simulink model "gm_uz_endat_interface_2025b"  (R2025b)
settings: Solver=FixedStepDiscrete  StartTime=0.0  StopTime=1.3e-3  RelTol=1e-3
undefined symbols (not defined in the file or in its folder): binary_or_gray, bit_sum, delay_first_clk_on_off, endat_clk_divider, endat_encoder_bit_width_multi_turn, endat_encoder_bit_width_single_turn, endat_encoder_number_of_CRC_bits, f_ADC, f_clock, PLL, t_ADC, t_clock, XData
libraries: hdlmdlgenlib x123, simulink x35, hdlsllib x29, simulink_extras x13
(part 3 of 4)

== system gm_uz_endat_interface_2025b/uz_endat_interface/position_to_speed_pll/Sine HDL Optimized1 ==
  u : Inport  OutDataTypeStr=fixdt(1, 27, 20)  SampleTime=1e-08
  sincos hdl : Subsystem  mask{NumDataPoints=256, TableDataTypeStr=fixdt(0,26,20), SimulateLUTROMDelay='Off'}
      mask prompts: NumDataPoints "HDLShared:hdlshared:CosineHDL_Npts"; TableDataTypeStr "Simulink:blkprm_prompts:TABLE_UNIFIEDDATATYPE"; SimulateLUTROMDelay "HDLShared:hdlshared:CosineHDL_SimulateLUTDelay"
      mask Display:
      | port_label('input',1,'u')
      | port_label('output',1,'sin(2*pi*u)')
      | port_label('output',2,'cos(2*pi*u)')
      | xpos = 0.35;
      | yoffset = 0.5;
      | if ( SimulateLUTROMDelay )
      |   text(xpos,yoffset,'HDL (Z^{-1})','texmode','on')
      | else
      |    text(xpos,yoffset,'HDL')
      | end
  x : Outport  SampleTime=1e-08  VectorParamsAs1DForOutWhenUnconnected=off
  y : Outport  Port=2  SampleTime=1e-08
  wires:
  u/1 -> sincos hdl/1(In1)
  sincos hdl/1(Out1) -> x/1
  sincos hdl/2(Out2) -> y/1

== system gm_uz_endat_interface_2025b/uz_endat_interface/position_to_speed_pll/fixed_point_floor ==
  x : Inport  OutDataTypeStr=fixdt(1, 27, 23)  PortDimensions=1  SampleTime=1e-08
  fixed_point_floor : MATLAB Function  TreatAsAtomicUnit=on
  y : Outport  SampleTime=1e-08  VectorParamsAs1DForOutWhenUnconnected=off
  wires:
  x/1 -> fixed_point_floor/1(x)
  fixed_point_floor/1(y) -> y/1

== system gm_uz_endat_interface_2025b/uz_endat_interface/serial_communication/MATLAB Function1 ==
  clocks : Inport  OutDataTypeStr=int32  PortDimensions=1  SampleTime=1e-08
  error1 : Inport  Port=2  OutDataTypeStr=uint32  PortDimensions=1  SampleTime=1e-08
  error2 : Inport  Port=3  OutDataTypeStr=uint32  PortDimensions=1  SampleTime=1e-08
  endat22 : Inport  Port=4  OutDataTypeStr=uint32  PortDimensions=1  SampleTime=1e-08
  highpos : Inport  Port=5  OutDataTypeStr=uint32  PortDimensions=1  SampleTime=1e-08
  lowpos : Inport  Port=6  OutDataTypeStr=uint32  PortDimensions=1  SampleTime=1e-08
  MATLAB Function1 : MATLAB Function  TreatAsAtomicUnit=on
  crc : Outport  SampleTime=1e-08  VectorParamsAs1DForOutWhenUnconnected=off
  wires:
  clocks/1 -> MATLAB Function1/1(clocks)
  error1/1 -> MATLAB Function1/2(error1)
  error2/1 -> MATLAB Function1/3(error2)
  endat22/1 -> MATLAB Function1/4(endat22)
  highpos/1 -> MATLAB Function1/5(highpos)
  MATLAB Function1/1(crc) -> crc/1
  lowpos/1 -> MATLAB Function1/6(lowpos)

== system gm_uz_endat_interface_2025b/uz_endat_interface/serial_communication/clk_idle_and_delay_first_clock_function ==
  note: U(k)
  note: Edge
  note: 194 equals 2.0µs
  delay_first_clk_on_off : Inport  OutDataTypeStr=boolean  PortDimensions=1  SampleTime=1e-08
  trigger_endat : Inport  Port=2  OutDataTypeStr=boolean  PortDimensions=1  SampleTime=1e-08
  endat_clk_enb_out : Inport  Port=3  OutDataTypeStr=boolean  PortDimensions=1  SampleTime=1e-08
  Constant4 : Constant  Value=0  OutDataTypeStr=boolean  SampleTime=1e-08
  Constant5 : Constant  OutDataTypeStr=boolean  SampleTime=1e-08
  Delay : Delay  DelayLength=double(194)  InitialCondition=0  SampleTime=1e-08
  Delay Input1 : UnitDelay  SampleTime=1e-08
  Delay1 : Delay  DelayLength=double(1)  InitialCondition=0  SampleTime=1e-08
  FixPt Relational Operator : RelationalOperator  Operator=>  OutDataTypeStr=boolean  SampleTime=1e-08  InputSameDT=off
  NOT : Logic  Operator=NOT  Inputs=1  AllPortsSameDT=off  OutDataTypeStr=boolean  SampleTime=1e-08
  Positive : simulink/Logic and Bit Operations/Compare To Constant  relop=>  const=double(0)  OutDataTypeStr=boolean
  S-R Flip-Flop : simulink_extras/Flip Flops/S-R Flip-Flop  initial_condition=0
  S-R Flip-Flop_inst_term1 : Terminator
  Switch : Switch  Criteria=u2 > Threshold  Threshold="fi(0,0,1,0,\"hex\",\"0\")"  OutDataTypeStr=boolean  SampleTime=1e-08  SaturateOnIntegerOverflow=off  InputSameDT=off
  Switch3 : Switch  Criteria=u2 > Threshold  Threshold="fi(0,0,1,0,\"hex\",\"0\")"  OutDataTypeStr=boolean  SampleTime=1e-08  SaturateOnIntegerOverflow=off  InputSameDT=off
  Switch4 : Switch  Criteria=u2 > Threshold  Threshold="fi(0,0,1,0,\"hex\",\"0\")"  OutDataTypeStr=boolean  SampleTime=1e-08  SaturateOnIntegerOverflow=off  InputSameDT=off
  endat_clk_enb : Outport  SampleTime=1e-08
  endat_clk_idle_levels : Outport  Port=2  SampleTime=1e-08
  wires:
  endat_clk_enb_out/1 -> NOT/1
  S-R Flip-Flop/1 -> Switch/2, Delay1/1, Delay/1
  NOT/1 -> Positive/1
  Positive/1 -> Delay Input1/1, FixPt Relational Operator/1
  FixPt Relational Operator/1 -> S-R Flip-Flop/2
  Delay Input1/1 -> FixPt Relational Operator/2
  S-R Flip-Flop/2 -> S-R Flip-Flop_inst_term1/1
  trigger_endat/1 -> S-R Flip-Flop/1
  Constant4/1 -> Switch/1
  Constant5/1 -> Switch/3
  Delay/1 -> Switch4/1
  Delay1/1 -> Switch4/2, Switch4/3, Switch3/3
  Switch/1 -> endat_clk_idle_levels/1
  Switch4/1 -> Switch3/1
  delay_first_clk_on_off/1 -> Switch3/2
  Switch3/1 -> endat_clk_enb/1

== system gm_uz_endat_interface_2025b/uz_endat_interface/serial_communication/endat_clock_enable_controller ==
  note: U(k)
  note: Edge
  note: U(k)
  note: Edge
  note: counter starts at 1, because the start-bit sets the SR flip-flop that allows for subsequent clk pulses to increment the counter. Since the start-bit is already the first bit we start with counter at 1 and the next rising edge of the clock increments to 2 which is the Fehler 1 bit
  endat_clk_enb_in : Inport  OutDataTypeStr=boolean  PortDimensions=1  SampleTime=1e-08
  max_num_of_clock_pulses_to_send : Inport  Port=2  OutDataTypeStr=uint32  PortDimensions=1  SampleTime=1e-08
  endat_clk_in : Inport  Port=3  OutDataTypeStr=boolean  PortDimensions=1  SampleTime=1e-08
  timeout_num_of_clock_pulses_to_send : Inport  Port=4  OutDataTypeStr=uint32  PortDimensions=1  SampleTime=1e-08
  start_bit_detected : Inport  Port=5  OutDataTypeStr=boolean  PortDimensions=1  SampleTime=1e-08
  AND1 : Logic  AllPortsSameDT=off  OutDataTypeStr=boolean  SampleTime=1e-08
  AND2 : Logic  AllPortsSameDT=off  OutDataTypeStr=boolean  SampleTime=1e-08
  Constant : Constant  Value=0  OutDataTypeStr=boolean  SampleTime=1e-08
  Constant1 : Constant  Value=2  OutDataTypeStr=uint8  SampleTime=1e-08
  Delay Input1 : UnitDelay  SampleTime=1e-08
  Delay Input11 : UnitDelay  SampleTime=1e-08
  FixPt Relational Operator : RelationalOperator  Operator=>  OutDataTypeStr=boolean  SampleTime=1e-08  InputSameDT=off
  FixPt Relational Operator1 : RelationalOperator  Operator=>  OutDataTypeStr=boolean  SampleTime=1e-08  InputSameDT=off
  HDL Counter : hdlsllib/Sources/HDL Counter  CountType=Free running  CountInit=0  CountStep=1  CountMax=25  CountFromType=Initial value  CountFrom=0  CountResetPort=on  CountLoadPort=off  CountEnbPort=on  CountDirPort=off  CountHitOutputPort=off  CountDataType=Unsigned  CountWordLen=8  CountFracLen=0  CountSampTime=1
  HDL Counter1 : hdlsllib/Sources/HDL Counter  CountType=Free running  CountInit=1  CountStep=1  CountMax=25  CountFromType=Initial value  CountFrom=1  CountResetPort=on  CountLoadPort=off  CountEnbPort=on  CountDirPort=off  CountHitOutputPort=off  CountDataType=Unsigned  CountWordLen=8  CountFracLen=0  CountSampTime=1
  OR : Logic  Operator=OR  AllPortsSameDT=off  OutDataTypeStr=boolean  SampleTime=1e-08
  Positive : simulink/Logic and Bit Operations/Compare To Constant  relop=>  const=double(0)  OutDataTypeStr=boolean
  Positive1 : simulink/Logic and Bit Operations/Compare To Constant  relop=>  const=double(0)  OutDataTypeStr=boolean
  Relational Operator : RelationalOperator  OutDataTypeStr=boolean  SampleTime=1e-08  InputSameDT=off
  Relational Operator1 : RelationalOperator  OutDataTypeStr=boolean  SampleTime=1e-08  InputSameDT=off
  Relational Operator2 : RelationalOperator  Operator=>  OutDataTypeStr=boolean  SampleTime=1e-08  InputSameDT=off
  S-R Flip-Flop : simulink_extras/Flip Flops/S-R Flip-Flop  initial_condition=0
  S-R Flip-Flop1 : simulink_extras/Flip Flops/S-R Flip-Flop  initial_condition=0
  S-R Flip-Flop1_inst_term1 : Terminator
  S-R Flip-Flop_inst_term1 : Terminator
  Switch : Switch  Criteria=u2 > Threshold  Threshold="fi(0,0,1,0,\"hex\",\"0\")"  OutDataTypeStr=boolean  SampleTime=1e-08  SaturateOnIntegerOverflow=off  InputSameDT=off
  endat_clk_enb_out : Outport  SampleTime=1e-08
  condition_for_start_sampling_position_data : Outport  Port=2  SampleTime=1e-08
  wires:
  Relational Operator/1 -> AND1/1
  endat_clk_in/1 -> Positive/1, Positive1/1
  max_num_of_clock_pulses_to_send/1 -> Relational Operator/2
  timeout_num_of_clock_pulses_to_send/1 -> Relational Operator1/2
  HDL Counter/1 -> Relational Operator1/1
  Positive1/1 -> FixPt Relational Operator1/1, Delay Input11/1
  Positive/1 -> FixPt Relational Operator/1, Delay Input1/1
  Relational Operator1/1 -> AND2/1
  Delay Input11/1 -> FixPt Relational Operator1/2
  Delay Input1/1 -> FixPt Relational Operator/2
  AND1/1 -> OR/2
  FixPt Relational Operator1/1 -> AND1/2, AND2/2
  AND2/1 -> OR/1
  FixPt Relational Operator/1 -> HDL Counter/2, Switch/1
  Constant1/1 -> Relational Operator2/2
  Constant/1 -> Switch/3
  OR/1 -> S-R Flip-Flop1/2, S-R Flip-Flop/2, HDL Counter1/1, HDL Counter/1
  endat_clk_enb_in/1 -> S-R Flip-Flop/1
  Switch/1 -> HDL Counter1/2
  start_bit_detected/1 -> S-R Flip-Flop1/1
  S-R Flip-Flop/2 -> S-R Flip-Flop_inst_term1/1
  S-R Flip-Flop/1 -> endat_clk_enb_out/1
  S-R Flip-Flop1/2 -> S-R Flip-Flop1_inst_term1/1
  S-R Flip-Flop1/1 -> Switch/2
  HDL Counter1/1 -> Relational Operator/1, Relational Operator2/1
  Relational Operator2/1 -> condition_for_start_sampling_position_data/1

== system gm_uz_endat_interface_2025b/uz_endat_interface/serial_communication/endat_clock_generator ==
  note: U(k)
  note: Edge
  endat_clk_divider : Inport  OutDataTypeStr=uint32  PortDimensions=1  SampleTime=1e-08
  endat_clk_reset : Inport  Port=2  OutDataTypeStr=boolean  PortDimensions=1  SampleTime=1e-08
  endat_clk_enb : Inport  Port=3  OutDataTypeStr=boolean  PortDimensions=1  SampleTime=1e-08
  AND : Logic  AllPortsSameDT=off  OutDataTypeStr=boolean  SampleTime=1e-08
  AND1 : Logic  AllPortsSameDT=off  OutDataTypeStr=boolean  SampleTime=1e-08
  Constant : Constant  OutDataTypeStr=uint16  SampleTime=1e-08
  Data Type Conversion : DataTypeConversion  OutDataTypeStr=uint16  SampleTime=1e-08  SaturateOnIntegerOverflow=off  RndMeth=Floor
  Delay : Delay  DelayLength=double(1)  InitialCondition=0  SampleTime=1e-08
  Delay Input1 : UnitDelay  SampleTime=1e-08
  Delay1 : Delay  DelayLength=double(1)  InitialCondition=0  SampleTime=1e-08
  FixPt Relational Operator : RelationalOperator  Operator=>  OutDataTypeStr=boolean  SampleTime=1e-08  InputSameDT=off
  OR : Logic  Operator=OR  AllPortsSameDT=off  OutDataTypeStr=boolean  SampleTime=1e-08
  Positive : simulink/Logic and Bit Operations/Compare To Constant  relop=>  const=double(0)  OutDataTypeStr=boolean
  Relational Operator : RelationalOperator  OutDataTypeStr=boolean  SampleTime=1e-08  InputSameDT=off
  S-R Flip-Flop1 : simulink_extras/Flip Flops/S-R Flip-Flop  initial_condition=0
  Sum : Sum  Inputs=+-  OutDataTypeStr=uint16  AccumDataTypeStr=uint16  SampleTime=1e-08
  base_counter : hdlsllib/Sources/HDL Counter  CountType=Free running  CountInit=0  CountStep=1  CountMax=199  CountFromType=Initial value  CountFrom=0  CountResetPort=on  CountLoadPort=off  CountEnbPort=on  CountDirPort=off  CountHitOutputPort=off  CountDataType=Unsigned  CountWordLen=16  CountFracLen=0  CountSampTime=1
  endat_clk : Outport  SampleTime=1e-08
  wires:
  endat_clk_reset/1 -> OR/2
  endat_clk_divider/1 -> Data Type Conversion/1
  Positive/1 -> FixPt Relational Operator/1, Delay Input1/1
  endat_clk_enb/1 -> base_counter/2
  Data Type Conversion/1 -> Sum/1
  Relational Operator/1 -> base_counter/1
  Constant/1 -> Sum/2
  base_counter/1 -> Positive/1, Relational Operator/1
  Sum/1 -> Relational Operator/2
  Delay Input1/1 -> FixPt Relational Operator/2
  S-R Flip-Flop1/2 -> Delay1/1
  S-R Flip-Flop1/1 -> Delay/1, endat_clk/1
  FixPt Relational Operator/1 -> AND1/2, AND/1
  AND/1 -> OR/1
  Delay1/1 -> AND1/1
  Delay/1 -> AND/2
  AND1/1 -> S-R Flip-Flop1/1
  OR/1 -> S-R Flip-Flop1/2

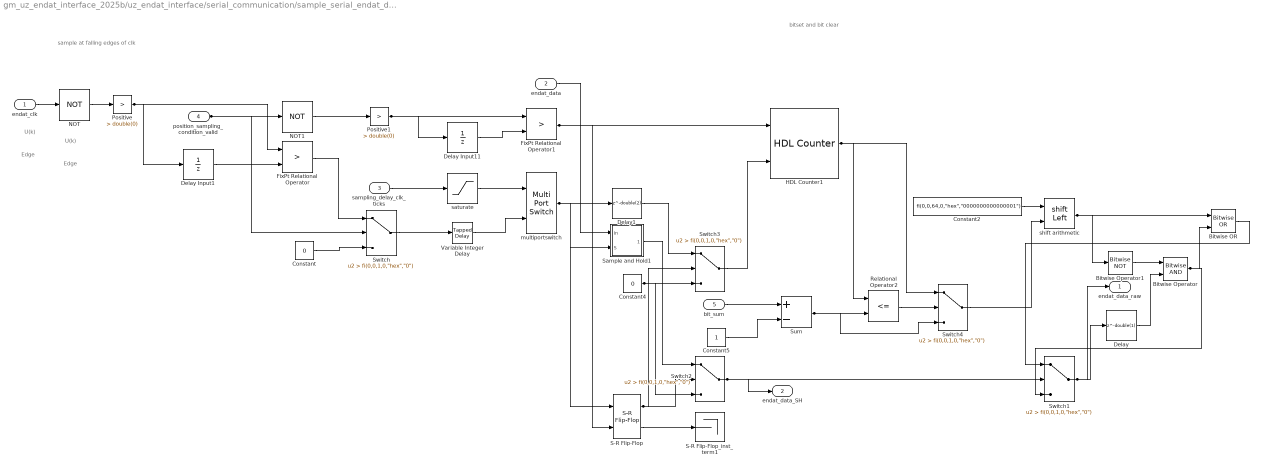
== system gm_uz_endat_interface_2025b/uz_endat_interface/serial_communication/sample_serial_endat_data ==
  note: U(k)
  note: Edge
  note: U(k)
  note: Edge
  note: sample at falling edges of clk
  note: bitset and bit clear
  endat_clk : Inport  OutDataTypeStr=boolean  PortDimensions=1  SampleTime=1e-08
  endat_data : Inport  Port=2  OutDataTypeStr=boolean  PortDimensions=1  SampleTime=1e-08
  sampling_delay_clk_ticks : Inport  Port=3  OutDataTypeStr=uint32  PortDimensions=1  SampleTime=1e-08
  position_sampling_condition_valid : Inport  Port=4  OutDataTypeStr=boolean  PortDimensions=1  SampleTime=1e-08
  bit_sum : Inport  Port=5  OutDataTypeStr=uint32  PortDimensions=1  SampleTime=1e-08
  Bitwise OR : simulink/Logic and Bit Operations/Bitwise Operator  logicop=OR  UseBitMask=off  NumInputPorts=2  BitMask=double(0)  BitMaskRealWorld=Real World Value
  Bitwise Operator : simulink/Logic and Bit Operations/Bitwise Operator  logicop=AND  UseBitMask=off  NumInputPorts=2  BitMask=double(0)  BitMaskRealWorld=Real World Value
  Bitwise Operator1 : simulink/Logic and Bit Operations/Bitwise Operator  logicop=NOT  UseBitMask=off  BitMask=double(0)  BitMaskRealWorld=Real World Value
  Constant : Constant  Value=0  OutDataTypeStr=boolean  SampleTime=1e-08
  Constant2 : Constant  Value="fi(0,0,64,0,\"hex\",\"0000000000000001\")"  OutDataTypeStr=fixdt(0, 64, 0)  SampleTime=1e-08
  Constant4 : Constant  Value=0  OutDataTypeStr=boolean  SampleTime=1e-08
  Constant5 : Constant  OutDataTypeStr=uint32  SampleTime=1e-08
  Delay : Delay  DelayLength=double(1)  InitialCondition=0  SampleTime=1e-08
  Delay Input1 : UnitDelay  SampleTime=1e-08
  Delay Input11 : UnitDelay  SampleTime=1e-08
  Delay1 : Delay  DelayLength=double(2)  InitialCondition=0  SampleTime=1e-08
  FixPt Relational Operator : RelationalOperator  Operator=>  OutDataTypeStr=boolean  SampleTime=1e-08  InputSameDT=off
  FixPt Relational Operator1 : RelationalOperator  Operator=>  OutDataTypeStr=boolean  SampleTime=1e-08  InputSameDT=off
  HDL Counter1 : hdlsllib/Sources/HDL Counter  CountType=Free running  CountInit=0  CountStep=1  CountMax=24  CountFromType=Initial value  CountFrom=0  CountResetPort=on  CountLoadPort=off  CountEnbPort=on  CountDirPort=off  CountHitOutputPort=off  CountDataType=Unsigned  CountWordLen=6  CountFracLen=0  CountSampTime=1
  NOT : Logic  Operator=NOT  Inputs=1  AllPortsSameDT=off  OutDataTypeStr=boolean  SampleTime=1e-08
  NOT1 : Logic  Operator=NOT  Inputs=1  AllPortsSameDT=off  OutDataTypeStr=boolean  SampleTime=1e-08
  Positive : simulink/Logic and Bit Operations/Compare To Constant  relop=>  const=double(0)  OutDataTypeStr=boolean
  Positive1 : simulink/Logic and Bit Operations/Compare To Constant  relop=>  const=double(0)  OutDataTypeStr=boolean
  Relational Operator2 : RelationalOperator  Operator=<=  OutDataTypeStr=boolean  SampleTime=1e-08  InputSameDT=off
  S-R Flip-Flop : simulink_extras/Flip Flops/S-R Flip-Flop  initial_condition=0
  S-R Flip-Flop_inst_term1 : Terminator
  Sample and Hold1 : Subsystem  mask(Sample and Hold){ic=double(0), Ts=double(1e-08)}
      mask prompts: ic "Initial condition:"; Ts "Sample time:"
      mask help:
      | Sample and hold input signal.
      |
      | The output follows input 1 (In) as long as input 2 (S) is TRUE (1). The output is held when input 2 becomes FALSE (0).
      mask init:
      | Ts = double(1e-08);
      | WantBlockChoice = 'Discrete';
      | block = 'uz_endat_interface_2025b/uz_endat_interface/serial_communication/sample_serial_endat_data/Sample and\nHold1';
      | ic = double(0);
      mask Help: helpview(psbhelp);
      mask Display: disp('S/H')
  Sum : Sum  Inputs=+-  OutDataTypeStr=uint32  AccumDataTypeStr=uint32  SampleTime=1e-08
  Switch : Switch  Criteria=u2 > Threshold  Threshold="fi(0,0,1,0,\"hex\",\"0\")"  OutDataTypeStr=boolean  SampleTime=1e-08  SaturateOnIntegerOverflow=off  InputSameDT=off
  Switch1 : Switch  Criteria=u2 > Threshold  Threshold="fi(0,0,1,0,\"hex\",\"0\")"  OutDataTypeStr=fixdt(0, 64, 0)  SampleTime=1e-08  SaturateOnIntegerOverflow=off  InputSameDT=off
  Switch2 : Switch  Criteria=u2 > Threshold  Threshold="fi(0,0,1,0,\"hex\",\"0\")"  OutDataTypeStr=boolean  SampleTime=1e-08  SaturateOnIntegerOverflow=off  InputSameDT=off
  Switch3 : Switch  Criteria=u2 > Threshold  Threshold="fi(0,0,1,0,\"hex\",\"0\")"  OutDataTypeStr=boolean  SampleTime=1e-08  SaturateOnIntegerOverflow=off  InputSameDT=off
  Switch4 : Switch  Criteria=u2 > Threshold  Threshold="fi(0,0,1,0,\"hex\",\"0\")"  OutDataTypeStr=uint32  SampleTime=1e-08  SaturateOnIntegerOverflow=off  InputSameDT=off
  Variable Integer Delay : simulink/Discrete/Tapped Delay  vinit=0  samptime=-1  NumDelays=double(100)  DelayOrder=Newest  includeCurrent=on
  multiportswitch : MultiPortSwitch  DataPortOrder=Zero-based contiguous  Inputs=1  DiagnosticForDefault=None  zeroidx=on  SampleTime=1e-08  SaturateOnIntegerOverflow=off  InputSameDT=off
  saturate : Saturate  UpperLimit=double(100)  LowerLimit=double(0)  SampleTime=1e-08  OutDataTypeStr=uint32
  shift arithmetic : ArithShift  BitShiftNumberSource=Input port  BitShiftDirection=Left
      settings: InputPortMap=u0,p1
  endat_data_raw : Outport  OutDataTypeStr=uint64  SampleTime=1e-08
  endat_data_SH : Outport  Port=2  SampleTime=1e-08
  wires:
  Constant/1 -> Switch/3
  endat_clk/1 -> NOT/1
  NOT/1 -> Positive/1
  sampling_delay_clk_ticks/1 -> saturate/1
  Positive/1 -> FixPt Relational Operator/1, Delay Input1/1
  bit_sum/1 -> Sum/1
  position_sampling_condition_valid/1 -> Switch/2, NOT1/1
  FixPt Relational Operator/1 -> Switch/1
  Delay Input1/1 -> FixPt Relational Operator/2
  NOT1/1 -> Positive1/1
  Positive1/1 -> FixPt Relational Operator1/1, Delay Input11/1
  Switch/1 -> Variable Integer Delay/1
  Delay Input11/1 -> FixPt Relational Operator1/2
  saturate/1 -> multiportswitch/1
  Delay1/1 -> Switch3/1
  Variable Integer Delay/1 -> multiportswitch/2
  endat_data/1 -> Sample and Hold1/1(In)
  FixPt Relational Operator1/1 -> HDL Counter1/1, S-R Flip-Flop/2
  multiportswitch/1 -> Delay1/1, Sample and Hold1/2(S), S-R Flip-Flop/1
  Sample and Hold1/1("   ") -> Switch2/1
  Bitwise OR/1 -> Switch1/1
  Constant4/1 -> Switch3/3, Switch2/3
  S-R Flip-Flop/2 -> S-R Flip-Flop_inst_term1/1
  S-R Flip-Flop/1 -> Switch3/2, Switch2/2
  Constant5/1 -> Sum/2
  Switch3/1 -> HDL Counter1/2
  Switch2/1 -> Switch1/2, endat_data_SH/1
  Relational Operator2/1 -> Switch4/2
  HDL Counter1/1 -> Switch4/1, Relational Operator2/1
  Sum/1 -> Relational Operator2/2, Switch4/3
  Constant2/1 -> shift arithmetic/1
  Switch4/1 -> shift arithmetic/2
  shift arithmetic/1 -> Bitwise OR/1, Bitwise Operator1/1
  Switch1/1 -> endat_data_raw/1, Delay/1
  Bitwise Operator1/1 -> Bitwise Operator/1
  Delay/1 -> Bitwise Operator/2
  Bitwise Operator/1 -> Switch1/3, Bitwise OR/2

== system gm_uz_endat_interface_2025b/uz_endat_interface/set_offset_to_raw_position_and_wrap/floor_div_pow2 ==
  dividend : Inport  OutDataTypeStr=fixdt(1, 64, 0)  PortDimensions=1  SampleTime=1e-08
  divisor_power_of_two_bits : Inport  Port=2  OutDataTypeStr=uint32  PortDimensions=1  SampleTime=1e-08
  AND2 : Logic  IconShape=distinctive  AllPortsSameDT=off  OutDataTypeStr=boolean
  Bitwise AND6 : simulink/Logic and Bit Operations/Bitwise Operator  logicop=AND  UseBitMask=off  NumInputPorts=2  BitMask=bin2dec('11011001')  BitMaskRealWorld=Stored Integer
      settings: LibrarySourceBlock=|
      | simulink/Quick Insert/Logic and Bit
      | Operations/Bitwise AND
  Constant : Constant  Value=0  OutDataTypeStr=int64  SampleTime=-1
  Relational Operator : RelationalOperator  Operator=<  OutDataTypeStr=boolean  RndMeth=Simplest  InputSameDT=off
  Relational Operator1 : RelationalOperator  Operator=~=  OutDataTypeStr=boolean  RndMeth=Simplest  InputSameDT=off
  Shift Arithmetic4 : ArithShift  BitShiftNumberSource=Input port  BitShiftNumber=8  BitShiftDirection=Right
      settings: InputPortMap=u0,p1
  Shift Arithmetic5 : ArithShift  BitShiftNumberSource=Input port  BitShiftNumber=8  BitShiftDirection=Left
      settings: InputPortMap=u0,p1
  Sum10 : Sum  Inputs=|+-  OutDataTypeStr=int64
  Sum9 : Sum  Inputs=|+-  OutDataTypeStr=int64
  Switch : Switch  Criteria=u2 > Threshold  OutDataTypeStr=fixdt(1, 64, 0)  SaturateOnIntegerOverflow=off  InputSameDT=off
  const4 : Constant  OutDataTypeStr=int64  SampleTime=t_clock
  quotient : Outport  SampleTime=1e-08
  wires:
  Relational Operator1/1 -> AND2/2
  Bitwise AND6/1 -> Relational Operator1/1
  Sum9/1 -> Bitwise AND6/2
  const4/1 -> Sum9/2, Sum10/2, Shift Arithmetic5/1
  Shift Arithmetic5/1 -> Sum9/1
  divisor_power_of_two_bits/1 -> Shift Arithmetic5/2, Shift Arithmetic4/2
  dividend/1 -> Relational Operator/1, Shift Arithmetic4/1, Bitwise AND6/1
  Shift Arithmetic4/1 -> Switch/3, Sum10/1
  Constant/1 -> Relational Operator1/2, Relational Operator/2
  Sum10/1 -> Switch/1
  AND2/1 -> Switch/2
  Relational Operator/1 -> AND2/1
  Switch/1 -> quotient/1

== system gm_uz_endat_interface_2025b/uz_endat_interface/wrap_2pi/fixed_point_floor ==
  x : Inport  OutDataTypeStr=fixdt(0, 27, 24)  PortDimensions=1  SampleTime=1e-08
  fixed_point_floor : MATLAB Function  TreatAsAtomicUnit=on
  y : Outport  SampleTime=1e-08  VectorParamsAs1DForOutWhenUnconnected=off
  wires:
  x/1 -> fixed_point_floor/1(x)
  fixed_point_floor/1(y) -> y/1

== system gm_uz_endat_interface_2025b/uz_endat_interface/position_to_speed_pll/Sine HDL Optimized/sincos hdl ==
  In1 : Inport  OutDataTypeStr=fixdt(1, 27, 20)  SampleTime=1e-08
  cos_hdl : Subsystem  mask{NumDataPoints=double(256), TableDataTypeStr=fixdt(0,26,20), SimulateLUTROMDelay=Off}
      mask prompts: NumDataPoints "HDLShared:hdlshared:CosineHDL_Npts"; TableDataTypeStr "Simulink:blkprm_prompts:TABLE_UNIFIEDDATATYPE"; SimulateLUTROMDelay "HDLShared:hdlshared:CosineHDL_SimulateLUTDelay"
      mask init:
      | InputWordLength = double(10);
      | NumDataPoints = double(256);
      | OutputFracLength = double(20);
      | OutputWordLength = double(27);
      | SampleTime = double(-1);
      | SimulateLUTROMDelay = double(0);
      | TableDataTypeStr = fixdt(0,26,20);
      | TableFracLength = double(20);
      | TableWordLength = double(26);
      | YData = reshape(double([0;0.0061358846491544753;0.012271538285719925;0.01840672990580482;0.024541228522912288;0.030674803176636626;0.036807222941358832;0.04293825693494082;0.049067674327418015;0.055195244349689941;0.061320736302208578;0.067443919563664051;0.073564563599667426;0.079682437971430126;0.085797312344439894;0.091908956497132724;0.098017140329560604;0.10412163387205459;0.11022220729388306;0.11631863091190475;0.1224106751992162;0.12849811079379317;0.13458070850712617;0.14065823933284921;0.14673047445536175;0.15279718525844344;0.15885814333386145;0.16491312048996992;0.17096188876030122;0.17700422041214875;0.18303988795514095;0.18906866414980619;0.19509032201612825;0.2011046348420919;0.20711137619221856;0.21311031991609136;0.2191012401568698;0.22508391135979283;0.23105810828067111;0.2370236059943672;0.24298017990326387;0.24892760574572015;0.25486565960451457;0.26079411791527551;0.26671275747489837;0.27262135544994898;0.27851968938505306;0.28440753721127188;0.29028467725446233;0.29615088824362379;0.30200594931922808;0.30784964004153487;0.31368174039889152;0.31950203081601569;0.32531029216226293;0.33110630575987643;0.33688985339222005;0.34266071731199438;0.34841868024943456;0.35416352542049034;0.35989503653498811;0.36561299780477385;0.37131719395183749;0.37700741021641826;0.38268343236508978;0.38834504669882625;0.3939920400610481;0.39962419984564679;0.40524131400498986;0.41084317105790391;0.41642956009763715;0.42200027079979968;0.42755509343028208;0.43309381885315196;0.43861623853852766;0.4441221445704292;0.44961132965460654;0.45508358712634384;0.46053871095824001;0.46597649576796618;0.47139673682599764;0.47679923006332209;0.48218377207912272;0.487550160148436;0.49289819222978404;0.49822766697278181;0.50353838372571758;0.50883014254310699;0.51410274419322166;0.51935599016558964;0.52458968267846895;0.52980362468629461;0.53499761988709715;0.54017147272989285;0.54532498842204646;0.55045797293660481;0.55557023301960218;0.56066157619733603;0.56573181078361312;0.57078074588696726;0.57580819141784534;0.58081395809576453;0.58579785745643886;0.59075970185887416;0.59569930449243336;0.60061647938386897;0.60551104140432555;0.61038280627630948;0.61523159058062682;0.6200572117632891;0.62485948814238634;0.62963823891492698;0.63439328416364549;0.63912444486377573;0.64383154288979139;0.64851440102211244;0.65317284295377676;0.65780669329707864;0.66241577759017178;0.66699992230363747;0.67155895484701833;0.67609270357531592;0.68060099779545302;0.68508366777270036;0.68954054473706683;0.69397146088965389;0.69837624940897292;0.7027547444572253;0.70710678118654746;0.71143219574521643;0.71573082528381859;0.72000250796138165;0.72424708295146689;0.7284643904482252;0.73265427167241282;0.73681656887736979;0.74095112535495911;0.74505778544146595;0.74913639452345926;0.75318679904361252;0.75720884650648457;0.76120238548426178;0.76516726562245896;0.76910333764557959;0.77301045336273688;0.77688846567323244;0.78073722857209438;0.78455659715557524;0.78834642762660623;0.79210657730021228;0.79583690460888357;0.79953726910790501;0.80320753148064483;0.80684755354379922;0.81045719825259477;0.8140363297059483;0.81758481315158371;0.82110251499110465;0.82458930278502529;0.8280450452577558;0.83146961230254524;0.83486287498638001;0.83822470555483797;0.84155497743689833;0.84485356524970701;0.84812034480329712;0.8513551931052652;0.85455798836540053;0.85772861000027212;0.86086693863776731;0.8639728561215867;0.86704624551569265;0.87008699110871135;0.87309497841829009;0.8760700941954066;0.87901222642863341;0.88192126434835494;0.88479709843093779;0.88763962040285393;0.89044872324475788;0.89322430119551532;0.89596624975618511;0.89867446569395382;0.90134884704602203;0.90398929312344334;0.90659570451491533;0.90916798309052238;0.91170603200542988;0.91420975570353069;0.9166790599210427;0.91911385169005777;0.9215140393420419;0.92387953251128674;0.92621024213831138;0.92850608047321559;0.93076696107898371;0.93299279883473885;0.9351835099389475;0.93733901191257496;0.93945922360218992;0.94154406518302081;0.94359345816196039;0.94560732538052128;0.94758559101774109;0.94952818059303667;0.95143502096900834;0.95330604035419375;0.95514116830577067;0.95694033573220894;0.9587034748958716;0.96043051941556579;0.96212140426904158;0.96377606579543984;0.9653944416976894;0.96697647104485207;0.96852209427441727;0.97003125319454397;0.97150389098625178;0.97293995220556007;0.97433938278557586;0.97570213003852857;0.97702814265775439;0.97831737071962765;0.97956976568544052;0.98078528040323043;0.98196386910955524;0.98310548743121629;0.98421009238692903;0.98527764238894122;0.98630809724459867;0.98730141815785843;0.98825756773074946;0.98917650996478101;0.99005821026229712;0.99090263542778001;0.99170975366909953;0.99247953459870997;0.9932119492347945;0.99390697000235606;0.99456457073425542;0.99518472667219682;0.99576741446765982;0.996312612182778;0.99682029929116567;0.99729045667869021;0.99772306664419164;0.99811811290014918;0.99847558057329477;0.99879545620517241;0.99907772775264536;0.99932238458834954;0.99952941750109314;0.99969881869620425;0.9998305817958234;0.9999247018391445;0.99998117528260111]), [1  256]);
      | block_name = 'uz_endat_interface_2025b/uz_endat_interface/position_to_speed_pll/Sine\nHDL Optimized/sincos hdl/cos_hdl';
      | gcb_lut = double(11605.000122070312);
      mask Display:
      | port_label('input',1,'u')
      | port_label('output',1,'cos(2*pi*u)')
      | xpos = 0.35;
      | yoffset = 0.5;
      | if ( SimulateLUTROMDelay )
      |   text(xpos,yoffset,'HDL (Z^{-1})','texmode','on')
      | else
      |    text(xpos,yoffset,'HDL')
      | end
  sin_hdl : Subsystem  mask{NumDataPoints=double(256), TableDataTypeStr=fixdt(0,26,20), SimulateLUTROMDelay=Off}
      mask prompts: NumDataPoints "HDLShared:hdlshared:CosineHDL_Npts"; TableDataTypeStr "Simulink:blkprm_prompts:TABLE_UNIFIEDDATATYPE"; SimulateLUTROMDelay "HDLShared:hdlshared:CosineHDL_SimulateLUTDelay"
      mask init:
      | InputWordLength = double(10);
      | NumDataPoints = double(256);
      | OutputFracLength = double(20);
      | OutputWordLength = double(27);
      | SampleTime = double(-1);
      | SimulateLUTROMDelay = double(0);
      | TableDataTypeStr = fixdt(0,26,20);
      | TableFracLength = double(20);
      | TableWordLength = double(26);
      | YData = reshape(double([0;0.0061358846491544753;0.012271538285719925;0.01840672990580482;0.024541228522912288;0.030674803176636626;0.036807222941358832;0.04293825693494082;0.049067674327418015;0.055195244349689941;0.061320736302208578;0.067443919563664051;0.073564563599667426;0.079682437971430126;0.085797312344439894;0.091908956497132724;0.098017140329560604;0.10412163387205459;0.11022220729388306;0.11631863091190475;0.1224106751992162;0.12849811079379317;0.13458070850712617;0.14065823933284921;0.14673047445536175;0.15279718525844344;0.15885814333386145;0.16491312048996992;0.17096188876030122;0.17700422041214875;0.18303988795514095;0.18906866414980619;0.19509032201612825;0.2011046348420919;0.20711137619221856;0.21311031991609136;0.2191012401568698;0.22508391135979283;0.23105810828067111;0.2370236059943672;0.24298017990326387;0.24892760574572015;0.25486565960451457;0.26079411791527551;0.26671275747489837;0.27262135544994898;0.27851968938505306;0.28440753721127188;0.29028467725446233;0.29615088824362379;0.30200594931922808;0.30784964004153487;0.31368174039889152;0.31950203081601569;0.32531029216226293;0.33110630575987643;0.33688985339222005;0.34266071731199438;0.34841868024943456;0.35416352542049034;0.35989503653498811;0.36561299780477385;0.37131719395183749;0.37700741021641826;0.38268343236508978;0.38834504669882625;0.3939920400610481;0.39962419984564679;0.40524131400498986;0.41084317105790391;0.41642956009763715;0.42200027079979968;0.42755509343028208;0.43309381885315196;0.43861623853852766;0.4441221445704292;0.44961132965460654;0.45508358712634384;0.46053871095824001;0.46597649576796618;0.47139673682599764;0.47679923006332209;0.48218377207912272;0.487550160148436;0.49289819222978404;0.49822766697278181;0.50353838372571758;0.50883014254310699;0.51410274419322166;0.51935599016558964;0.52458968267846895;0.52980362468629461;0.53499761988709715;0.54017147272989285;0.54532498842204646;0.55045797293660481;0.55557023301960218;0.56066157619733603;0.56573181078361312;0.57078074588696726;0.57580819141784534;0.58081395809576453;0.58579785745643886;0.59075970185887416;0.59569930449243336;0.60061647938386897;0.60551104140432555;0.61038280627630948;0.61523159058062682;0.6200572117632891;0.62485948814238634;0.62963823891492698;0.63439328416364549;0.63912444486377573;0.64383154288979139;0.64851440102211244;0.65317284295377676;0.65780669329707864;0.66241577759017178;0.66699992230363747;0.67155895484701833;0.67609270357531592;0.68060099779545302;0.68508366777270036;0.68954054473706683;0.69397146088965389;0.69837624940897292;0.7027547444572253;0.70710678118654746;0.71143219574521643;0.71573082528381859;0.72000250796138165;0.72424708295146689;0.7284643904482252;0.73265427167241282;0.73681656887736979;0.74095112535495911;0.74505778544146595;0.74913639452345926;0.75318679904361252;0.75720884650648457;0.76120238548426178;0.76516726562245896;0.76910333764557959;0.77301045336273688;0.77688846567323244;0.78073722857209438;0.78455659715557524;0.78834642762660623;0.79210657730021228;0.79583690460888357;0.79953726910790501;0.80320753148064483;0.80684755354379922;0.81045719825259477;0.8140363297059483;0.81758481315158371;0.82110251499110465;0.82458930278502529;0.8280450452577558;0.83146961230254524;0.83486287498638001;0.83822470555483797;0.84155497743689833;0.84485356524970701;0.84812034480329712;0.8513551931052652;0.85455798836540053;0.85772861000027212;0.86086693863776731;0.8639728561215867;0.86704624551569265;0.87008699110871135;0.87309497841829009;0.8760700941954066;0.87901222642863341;0.88192126434835494;0.88479709843093779;0.88763962040285393;0.89044872324475788;0.89322430119551532;0.89596624975618511;0.89867446569395382;0.90134884704602203;0.90398929312344334;0.90659570451491533;0.90916798309052238;0.91170603200542988;0.91420975570353069;0.9166790599210427;0.91911385169005777;0.9215140393420419;0.92387953251128674;0.92621024213831138;0.92850608047321559;0.93076696107898371;0.93299279883473885;0.9351835099389475;0.93733901191257496;0.93945922360218992;0.94154406518302081;0.94359345816196039;0.94560732538052128;0.94758559101774109;0.94952818059303667;0.95143502096900834;0.95330604035419375;0.95514116830577067;0.95694033573220894;0.9587034748958716;0.96043051941556579;0.96212140426904158;0.96377606579543984;0.9653944416976894;0.96697647104485207;0.96852209427441727;0.97003125319454397;0.97150389098625178;0.97293995220556007;0.97433938278557586;0.97570213003852857;0.97702814265775439;0.97831737071962765;0.97956976568544052;0.98078528040323043;0.98196386910955524;0.98310548743121629;0.98421009238692903;0.98527764238894122;0.98630809724459867;0.98730141815785843;0.98825756773074946;0.98917650996478101;0.99005821026229712;0.99090263542778001;0.99170975366909953;0.99247953459870997;0.9932119492347945;0.99390697000235606;0.99456457073425542;0.99518472667219682;0.99576741446765982;0.996312612182778;0.99682029929116567;0.99729045667869021;0.99772306664419164;0.99811811290014918;0.99847558057329477;0.99879545620517241;0.99907772775264536;0.99932238458834954;0.99952941750109314;0.99969881869620425;0.9998305817958234;0.9999247018391445;0.99998117528260111]), [1  256]);
      | block_name = 'uz_endat_interface_2025b/uz_endat_interface/position_to_speed_pll/Sine\nHDL Optimized/sincos hdl/sin_hdl';
      | gcb_lut = double(11749.000122070312);
      mask Display:
      | port_label('input',1,'u')
      | port_label('output',1,'sin(2*pi*u)')
      | xpos = 0.35;
      | yoffset = 0.5;
      | if ( SimulateLUTROMDelay )
      |   text(xpos,yoffset,'HDL (Z^{-1})','texmode','on')
      | else
      |    text(xpos,yoffset,'HDL')
      | end
  Out1 : Outport  SampleTime=1e-08  VectorParamsAs1DForOutWhenUnconnected=off
  Out2 : Outport  Port=2  SampleTime=1e-08  VectorParamsAs1DForOutWhenUnconnected=off
  wires:
  In1/1 -> cos_hdl/1(In1), sin_hdl/1(In1)
  sin_hdl/1(y) -> Out1/1
  cos_hdl/1(x) -> Out2/1

== system gm_uz_endat_interface_2025b/uz_endat_interface/position_to_speed_pll/Sine HDL Optimized1/sincos hdl ==
  In1 : Inport  OutDataTypeStr=fixdt(1, 27, 20)  SampleTime=1e-08
  cos_hdl : Subsystem  mask{NumDataPoints=double(256), TableDataTypeStr=fixdt(0,26,20), SimulateLUTROMDelay=Off}
      mask prompts: NumDataPoints "HDLShared:hdlshared:CosineHDL_Npts"; TableDataTypeStr "Simulink:blkprm_prompts:TABLE_UNIFIEDDATATYPE"; SimulateLUTROMDelay "HDLShared:hdlshared:CosineHDL_SimulateLUTDelay"
      mask init:
      | InputWordLength = double(10);
      | NumDataPoints = double(256);
      | OutputFracLength = double(20);
      | OutputWordLength = double(27);
      | SampleTime = double(-1);
      | SimulateLUTROMDelay = double(0);
      | TableDataTypeStr = fixdt(0,26,20);
      | TableFracLength = double(20);
      | TableWordLength = double(26);
      | YData = reshape(double([0;0.0061358846491544753;0.012271538285719925;0.01840672990580482;0.024541228522912288;0.030674803176636626;0.036807222941358832;0.04293825693494082;0.049067674327418015;0.055195244349689941;0.061320736302208578;0.067443919563664051;0.073564563599667426;0.079682437971430126;0.085797312344439894;0.091908956497132724;0.098017140329560604;0.10412163387205459;0.11022220729388306;0.11631863091190475;0.1224106751992162;0.12849811079379317;0.13458070850712617;0.14065823933284921;0.14673047445536175;0.15279718525844344;0.15885814333386145;0.16491312048996992;0.17096188876030122;0.17700422041214875;0.18303988795514095;0.18906866414980619;0.19509032201612825;0.2011046348420919;0.20711137619221856;0.21311031991609136;0.2191012401568698;0.22508391135979283;0.23105810828067111;0.2370236059943672;0.24298017990326387;0.24892760574572015;0.25486565960451457;0.26079411791527551;0.26671275747489837;0.27262135544994898;0.27851968938505306;0.28440753721127188;0.29028467725446233;0.29615088824362379;0.30200594931922808;0.30784964004153487;0.31368174039889152;0.31950203081601569;0.32531029216226293;0.33110630575987643;0.33688985339222005;0.34266071731199438;0.34841868024943456;0.35416352542049034;0.35989503653498811;0.36561299780477385;0.37131719395183749;0.37700741021641826;0.38268343236508978;0.38834504669882625;0.3939920400610481;0.39962419984564679;0.40524131400498986;0.41084317105790391;0.41642956009763715;0.42200027079979968;0.42755509343028208;0.43309381885315196;0.43861623853852766;0.4441221445704292;0.44961132965460654;0.45508358712634384;0.46053871095824001;0.46597649576796618;0.47139673682599764;0.47679923006332209;0.48218377207912272;0.487550160148436;0.49289819222978404;0.49822766697278181;0.50353838372571758;0.50883014254310699;0.51410274419322166;0.51935599016558964;0.52458968267846895;0.52980362468629461;0.53499761988709715;0.54017147272989285;0.54532498842204646;0.55045797293660481;0.55557023301960218;0.56066157619733603;0.56573181078361312;0.57078074588696726;0.57580819141784534;0.58081395809576453;0.58579785745643886;0.59075970185887416;0.59569930449243336;0.60061647938386897;0.60551104140432555;0.61038280627630948;0.61523159058062682;0.6200572117632891;0.62485948814238634;0.62963823891492698;0.63439328416364549;0.63912444486377573;0.64383154288979139;0.64851440102211244;0.65317284295377676;0.65780669329707864;0.66241577759017178;0.66699992230363747;0.67155895484701833;0.67609270357531592;0.68060099779545302;0.68508366777270036;0.68954054473706683;0.69397146088965389;0.69837624940897292;0.7027547444572253;0.70710678118654746;0.71143219574521643;0.71573082528381859;0.72000250796138165;0.72424708295146689;0.7284643904482252;0.73265427167241282;0.73681656887736979;0.74095112535495911;0.74505778544146595;0.74913639452345926;0.75318679904361252;0.75720884650648457;0.76120238548426178;0.76516726562245896;0.76910333764557959;0.77301045336273688;0.77688846567323244;0.78073722857209438;0.78455659715557524;0.78834642762660623;0.79210657730021228;0.79583690460888357;0.79953726910790501;0.80320753148064483;0.80684755354379922;0.81045719825259477;0.8140363297059483;0.81758481315158371;0.82110251499110465;0.82458930278502529;0.8280450452577558;0.83146961230254524;0.83486287498638001;0.83822470555483797;0.84155497743689833;0.84485356524970701;0.84812034480329712;0.8513551931052652;0.85455798836540053;0.85772861000027212;0.86086693863776731;0.8639728561215867;0.86704624551569265;0.87008699110871135;0.87309497841829009;0.8760700941954066;0.87901222642863341;0.88192126434835494;0.88479709843093779;0.88763962040285393;0.89044872324475788;0.89322430119551532;0.89596624975618511;0.89867446569395382;0.90134884704602203;0.90398929312344334;0.90659570451491533;0.90916798309052238;0.91170603200542988;0.91420975570353069;0.9166790599210427;0.91911385169005777;0.9215140393420419;0.92387953251128674;0.92621024213831138;0.92850608047321559;0.93076696107898371;0.93299279883473885;0.9351835099389475;0.93733901191257496;0.93945922360218992;0.94154406518302081;0.94359345816196039;0.94560732538052128;0.94758559101774109;0.94952818059303667;0.95143502096900834;0.95330604035419375;0.95514116830577067;0.95694033573220894;0.9587034748958716;0.96043051941556579;0.96212140426904158;0.96377606579543984;0.9653944416976894;0.96697647104485207;0.96852209427441727;0.97003125319454397;0.97150389098625178;0.97293995220556007;0.97433938278557586;0.97570213003852857;0.97702814265775439;0.97831737071962765;0.97956976568544052;0.98078528040323043;0.98196386910955524;0.98310548743121629;0.98421009238692903;0.98527764238894122;0.98630809724459867;0.98730141815785843;0.98825756773074946;0.98917650996478101;0.99005821026229712;0.99090263542778001;0.99170975366909953;0.99247953459870997;0.9932119492347945;0.99390697000235606;0.99456457073425542;0.99518472667219682;0.99576741446765982;0.996312612182778;0.99682029929116567;0.99729045667869021;0.99772306664419164;0.99811811290014918;0.99847558057329477;0.99879545620517241;0.99907772775264536;0.99932238458834954;0.99952941750109314;0.99969881869620425;0.9998305817958234;0.9999247018391445;0.99998117528260111]), [1  256]);
      | block_name = 'uz_endat_interface_2025b/uz_endat_interface/position_to_speed_pll/Sine\nHDL Optimized1/sincos hdl/cos_hdl';
      | gcb_lut = double(12589.000366210938);
      mask Display:
      | port_label('input',1,'u')
      | port_label('output',1,'cos(2*pi*u)')
      | xpos = 0.35;
      | yoffset = 0.5;
      | if ( SimulateLUTROMDelay )
      |   text(xpos,yoffset,'HDL (Z^{-1})','texmode','on')
      | else
      |    text(xpos,yoffset,'HDL')
      | end
  sin_hdl : Subsystem  mask{NumDataPoints=double(256), TableDataTypeStr=fixdt(0,26,20), SimulateLUTROMDelay=Off}
      mask prompts: NumDataPoints "HDLShared:hdlshared:CosineHDL_Npts"; TableDataTypeStr "Simulink:blkprm_prompts:TABLE_UNIFIEDDATATYPE"; SimulateLUTROMDelay "HDLShared:hdlshared:CosineHDL_SimulateLUTDelay"
      mask init:
      | InputWordLength = double(10);
      | NumDataPoints = double(256);
      | OutputFracLength = double(20);
      | OutputWordLength = double(27);
      | SampleTime = double(-1);
      | SimulateLUTROMDelay = double(0);
      | TableDataTypeStr = fixdt(0,26,20);
      | TableFracLength = double(20);
      | TableWordLength = double(26);
      | YData = reshape(double([0;0.0061358846491544753;0.012271538285719925;0.01840672990580482;0.024541228522912288;0.030674803176636626;0.036807222941358832;0.04293825693494082;0.049067674327418015;0.055195244349689941;0.061320736302208578;0.067443919563664051;0.073564563599667426;0.079682437971430126;0.085797312344439894;0.091908956497132724;0.098017140329560604;0.10412163387205459;0.11022220729388306;0.11631863091190475;0.1224106751992162;0.12849811079379317;0.13458070850712617;0.14065823933284921;0.14673047445536175;0.15279718525844344;0.15885814333386145;0.16491312048996992;0.17096188876030122;0.17700422041214875;0.18303988795514095;0.18906866414980619;0.19509032201612825;0.2011046348420919;0.20711137619221856;0.21311031991609136;0.2191012401568698;0.22508391135979283;0.23105810828067111;0.2370236059943672;0.24298017990326387;0.24892760574572015;0.25486565960451457;0.26079411791527551;0.26671275747489837;0.27262135544994898;0.27851968938505306;0.28440753721127188;0.29028467725446233;0.29615088824362379;0.30200594931922808;0.30784964004153487;0.31368174039889152;0.31950203081601569;0.32531029216226293;0.33110630575987643;0.33688985339222005;0.34266071731199438;0.34841868024943456;0.35416352542049034;0.35989503653498811;0.36561299780477385;0.37131719395183749;0.37700741021641826;0.38268343236508978;0.38834504669882625;0.3939920400610481;0.39962419984564679;0.40524131400498986;0.41084317105790391;0.41642956009763715;0.42200027079979968;0.42755509343028208;0.43309381885315196;0.43861623853852766;0.4441221445704292;0.44961132965460654;0.45508358712634384;0.46053871095824001;0.46597649576796618;0.47139673682599764;0.47679923006332209;0.48218377207912272;0.487550160148436;0.49289819222978404;0.49822766697278181;0.50353838372571758;0.50883014254310699;0.51410274419322166;0.51935599016558964;0.52458968267846895;0.52980362468629461;0.53499761988709715;0.54017147272989285;0.54532498842204646;0.55045797293660481;0.55557023301960218;0.56066157619733603;0.56573181078361312;0.57078074588696726;0.57580819141784534;0.58081395809576453;0.58579785745643886;0.59075970185887416;0.59569930449243336;0.60061647938386897;0.60551104140432555;0.61038280627630948;0.61523159058062682;0.6200572117632891;0.62485948814238634;0.62963823891492698;0.63439328416364549;0.63912444486377573;0.64383154288979139;0.64851440102211244;0.65317284295377676;0.65780669329707864;0.66241577759017178;0.66699992230363747;0.67155895484701833;0.67609270357531592;0.68060099779545302;0.68508366777270036;0.68954054473706683;0.69397146088965389;0.69837624940897292;0.7027547444572253;0.70710678118654746;0.71143219574521643;0.71573082528381859;0.72000250796138165;0.72424708295146689;0.7284643904482252;0.73265427167241282;0.73681656887736979;0.74095112535495911;0.74505778544146595;0.74913639452345926;0.75318679904361252;0.75720884650648457;0.76120238548426178;0.76516726562245896;0.76910333764557959;0.77301045336273688;0.77688846567323244;0.78073722857209438;0.78455659715557524;0.78834642762660623;0.79210657730021228;0.79583690460888357;0.79953726910790501;0.80320753148064483;0.80684755354379922;0.81045719825259477;0.8140363297059483;0.81758481315158371;0.82110251499110465;0.82458930278502529;0.8280450452577558;0.83146961230254524;0.83486287498638001;0.83822470555483797;0.84155497743689833;0.84485356524970701;0.84812034480329712;0.8513551931052652;0.85455798836540053;0.85772861000027212;0.86086693863776731;0.8639728561215867;0.86704624551569265;0.87008699110871135;0.87309497841829009;0.8760700941954066;0.87901222642863341;0.88192126434835494;0.88479709843093779;0.88763962040285393;0.89044872324475788;0.89322430119551532;0.89596624975618511;0.89867446569395382;0.90134884704602203;0.90398929312344334;0.90659570451491533;0.90916798309052238;0.91170603200542988;0.91420975570353069;0.9166790599210427;0.91911385169005777;0.9215140393420419;0.92387953251128674;0.92621024213831138;0.92850608047321559;0.93076696107898371;0.93299279883473885;0.9351835099389475;0.93733901191257496;0.93945922360218992;0.94154406518302081;0.94359345816196039;0.94560732538052128;0.94758559101774109;0.94952818059303667;0.95143502096900834;0.95330604035419375;0.95514116830577067;0.95694033573220894;0.9587034748958716;0.96043051941556579;0.96212140426904158;0.96377606579543984;0.9653944416976894;0.96697647104485207;0.96852209427441727;0.97003125319454397;0.97150389098625178;0.97293995220556007;0.97433938278557586;0.97570213003852857;0.97702814265775439;0.97831737071962765;0.97956976568544052;0.98078528040323043;0.98196386910955524;0.98310548743121629;0.98421009238692903;0.98527764238894122;0.98630809724459867;0.98730141815785843;0.98825756773074946;0.98917650996478101;0.99005821026229712;0.99090263542778001;0.99170975366909953;0.99247953459870997;0.9932119492347945;0.99390697000235606;0.99456457073425542;0.99518472667219682;0.99576741446765982;0.996312612182778;0.99682029929116567;0.99729045667869021;0.99772306664419164;0.99811811290014918;0.99847558057329477;0.99879545620517241;0.99907772775264536;0.99932238458834954;0.99952941750109314;0.99969881869620425;0.9998305817958234;0.9999247018391445;0.99998117528260111]), [1  256]);
      | block_name = 'uz_endat_interface_2025b/uz_endat_interface/position_to_speed_pll/Sine\nHDL Optimized1/sincos hdl/sin_hdl';
      | gcb_lut = double(12736.000122070312);
      mask Display:
      | port_label('input',1,'u')
      | port_label('output',1,'sin(2*pi*u)')
      | xpos = 0.35;
      | yoffset = 0.5;
      | if ( SimulateLUTROMDelay )
      |   text(xpos,yoffset,'HDL (Z^{-1})','texmode','on')
      | else
      |    text(xpos,yoffset,'HDL')
      | end
  Out1 : Outport  SampleTime=1e-08  VectorParamsAs1DForOutWhenUnconnected=off
  Out2 : Outport  Port=2  SampleTime=1e-08  VectorParamsAs1DForOutWhenUnconnected=off
  wires:
  sin_hdl/1(y) -> Out1/1
  In1/1 -> cos_hdl/1(In1), sin_hdl/1(In1)
  cos_hdl/1(x) -> Out2/1

== system gm_uz_endat_interface_2025b/uz_endat_interface/serial_communication/sample_serial_endat_data/Sample and Hold1 ==
  In : Inport  OutDataTypeStr=boolean  SampleTime=1e-08
  S : Inport  Port=2  OutDataTypeStr=boolean  SampleTime=1e-08
  Model : Subsystem
  "   " : Outport  SampleTime=1e-08  InitialOutput=0  VectorParamsAs1DForOutWhenUnconnected=off
  wires:
  In/1 -> Model/1(In)
  S/1 -> Model/2(S)
  Model/1(Out) -> "   "/1
